simulink model "LoadCell"  (R2025a)
settings: Solver=FixedStepAuto  StartTime=0.0  StopTime=inf  RelTol=1e-3  EnableMultiTasking=on
undefined symbols (not defined in the file or in its folder): dspblkCoreblockFVToolHelper, gcbh
libraries: stm32f4xxblockslib x1, dspsnks4 x1, dspfiltersrcs x1, dspstat3 x1
settings Model: STM32="{\"AnalogInput\":[{\"ID\":\"untitled:1\"},{\"ID\":\"LoadCell:1\"}]}"  Creator=rajap  LastModifiedBy=rajap
settings OptimizationCC: DefaultParameterBehavior=Inlined  EnhancedBackFolding=on  PassReuseOutputArgsAs=Individual arguments  ZeroExternalMemoryAtStartup=off  ZeroInternalMemoryAtStartup=off  MaxStackSize=512  OptimizeBlockOrder=speed  DifferentSizesBufferReuse=on  OptimizationCustomize=off  EfficientTunableParamExpr=on
settings DebuggingCC: ParameterTunabilityLossMsg=error
settings HardwareCC: ProdBitPerPointer=32.0  ProdBitPerSizeT=32.0  ProdBitPerPtrDiffT=32.0  ProdLargestAtomicInteger=Long  ProdLargestAtomicFloat=Double  ProdWordSize=32.0  ProdLongLongMode=on  ProdHWDeviceType=ARM Compatible->ARM Cortex-M
settings SFSimCC: MATLABDynamicMemAlloc=off
settings RTWCC: SystemTargetFile=ert.tlc  HardwareBoard=STM32G4xx Based  TemplateMakefile=ert_default_tmf  Toolchain=GNU Tools for ARM Embedded Processors  Description=Embedded Coder
settings CodeAppCC: ForceParamTrailComments=on  IgnoreCustomStorageClasses=off  OperatorAnnotations=on  SimulinkDataObjDesc=on  SFDataObjDesc=on  InsertBlockDesc=on
settings ERTTargetCC: ExtModeTransport=3.0  ExtModeStaticAllocSize=2048.0  TargetLangStandard=C99 (ISO)  CodeReplacementLibrary=ARM Cortex-M

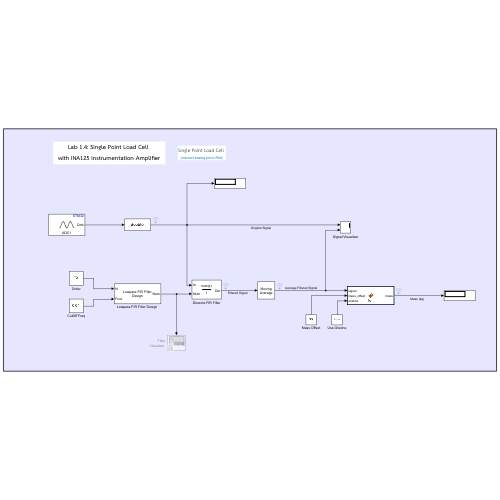
[thumbnail: Simulink's stored preview of the top-level diagram]
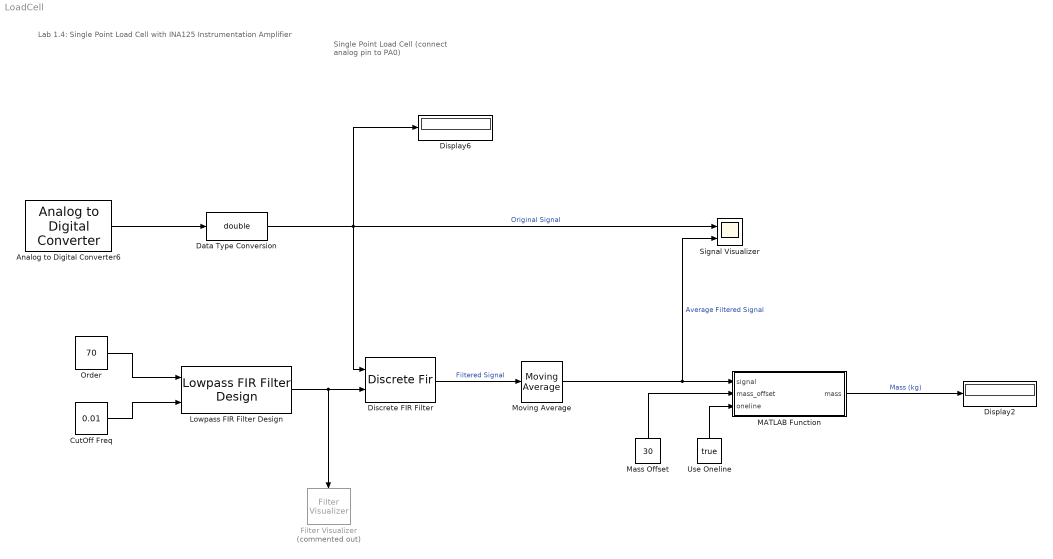
== system LoadCell ==
  note: Single Point Load Cell
      | (connect analog pin to PA0)
  note: Lab 1.4: Single Point Load Cell
      | with INA125 Instrumentation Amplifier
  Analog to Digital Converter6 : stm32f4xxblockslib/Analog to Digital Converter  ADCModule=ADC1  ConversionGroup=Regular  TriggerMode=Trigger and read  NumberOfConversions=1  EnableBufferConv=off  BufferLength=1  OutputStatus=off  SampleTime=-1  EnableSimPort=off  hoistedMaskSrc=ECSoC/ECSimCodegen/Analog to Digital Converter
  CutOff Freq : Constant  Value=0.01  VectorParams1D=off  SampleTime=-1
  Data Type Conversion : DataTypeConversion  OutDataTypeStr=double  SaturateOnIntegerOverflow=off  RndMeth=Floor
  Discrete FIR Filter : DiscreteFir  LoadFcn=dspblkCoreblockFVToolHelper(gcbh,'load');  CoefSource=Input port
      settings: CopyFcn=dspblkCoreblockFVToolHelper(gcbh,'copy');  DeleteFcn=dspblkCoreblockFVToolHelper(gcbh,'close');  ModelCloseFcn=dspblkCoreblockFVToolHelper(gcbh,'close');  PreSaveFcn=dspblkCoreblockFVToolHelper(gcbh,'presave');  PostSaveFcn=dspblkCoreblockFVToolHelper(gcbh,'postsave');  CloseFcn=dspblkCoreblockFVToolHelper(gcbh,'close');  InputPortMap=u0,u1
  Display2 : Display
  Display6 : Display
  "Filter Visualizer " : dspsnks4/Filter Visualizer  Commented=on  NumFilters=1  FilterType=FIR  FFTLength=2048  NormalizedFrequency=on  SampleRate=44100  FrequencyRange=[0,1]  XScale=Linear  MagnitudeDisplay=Magnitude (dB)  PlotAsMagnitudePhase=off  PlotType=Line  AxesScaling=Auto  AxesScalingNumUpdates=100  MaximizeAxes=Auto  Title=Magnitude Response  YLimits=[-154.01502622135783 48.12265248858887]  ShowLegend=off  FilterNames=[]  ShowGrid=on  Visible=off  ExpandToolstrip=off
  "Lowpass FIR Filter Design " : dspfiltersrcs/Lowpass FIR Filter Design  SmoothParameters=off  SmoothingFactor=0.6  FilterOrderPort=on  FilterOrder=100  MaxOrder=100  CutoffFrequencyPort=on  CutoffFrequency=0.01  Window=Hamming  SidelobeAttenuationPort=off  SidelobeAttenuation=60  KaiserWindowParameterPort=off  KaiserWindowParameter=.5  OutputDataType=double  SampleTime=-1  SimulateUsing=Interpreted execution
      settings: LibrarySourceBlock=dspfdesign/Lowpass FIR Filter Design
  MATLAB Function : MATLAB Function  TreatAsAtomicUnit=on
  Mass Offset : Constant  Value=30
  Moving Average : dspstat3/Moving Average  Method=Sliding window  ForgettingFactorPort=off  SpecifyWindowLength=on  WindowLength=100  OverlapLength=99  AllowArbitraryInputLength=off  ForgettingFactor=0.9  SimulateUsing=Interpreted execution
  Order : Constant  Value=70  VectorParams1D=off  SampleTime=-1
  Signal Visualizer : Scope  NumInputPorts=2
      settings: ActiveDisplayYMinimum=-334.16409269377715  ActiveDisplayYMaximum=280.92841792775408  DataLoggingVariableName=ScopeData2  DataLoggingSaveFormat=Array
  Use Oneline : Constant  Value=true
  wires:
  Order/1 -> "Lowpass FIR Filter Design "/1
  CutOff Freq/1 -> "Lowpass FIR Filter Design "/2
  Discrete FIR Filter/1 -> Moving Average/1  "Filtered Signal"
  MATLAB Function/1(mass) -> Display2/1  "Mass (kg)"
  Mass Offset/1 -> MATLAB Function/2(mass_offset)
  Data Type Conversion/1 -> Signal Visualizer/1, Display6/1, Discrete FIR Filter/1  "Original Signal"
  "Lowpass FIR Filter Design "/1 -> Discrete FIR Filter/2, "Filter Visualizer "/1
  Analog to Digital Converter6/1 -> Data Type Conversion/1
  Moving Average/1 -> Signal Visualizer/2, MATLAB Function/1(signal)  "Average Filtered Signal"
  Use Oneline/1 -> MATLAB Function/3(oneline)

== matlab function LoadCell/MATLAB Function ==
  data: signal input; mass output; mass_offset input; oneline input
function mass = fcn(signal, mass_offset, oneline)

if oneline
    mass = 3.178026669113850E+00*signal - 1.168297969921710E+02;
else
    if signal < 970
        mass = -1.352093207936490E-14*signal^6 + 4.432131629887790E-11*signal^5 - 5.738741720106180E-08*signal^4 + 3.737936611475020E-05*signal^3 - 1.297904608080040E-02*signal^2 + 5.576169021073690E+00*signal - 3.038874724538260E+02;
    else
        if signal <= 2248
            mass = 1.550683908461470E-16*signal^6 - 1.484162100433210E-12*signal^5 + 5.760240231668440E-09*signal^4 - 1.155867381281470E-05*signal^3 + 1.260145589933000E-02*signal^2 - 3.935837313266380E+00*signal + 1.557185519735790E+03;
        else
            mass = 5.323006496834790E-14*signal^6 - 8.394282399266000E-10*signal^5 + 5.504217910195670E-06*signal^4 - 1.920878746001660E-02*signal^3 + 3.762860391575460E+01*signal^2 - 3.922742305098780E+04*signal + 1.700615936684920E+07;
        end
    end
end

mass = mass - mass_offset;
if mass < 0
    mass = 0;
end

mass = mass/1000;

end
